simulink model "zadatak1"  (R2017b)
settings: Solver=VariableStepAuto  StartTime=0.0  StopTime=10.0  RelTol=1e-3
settings Model: Creator=HP  LastModifiedBy=HP

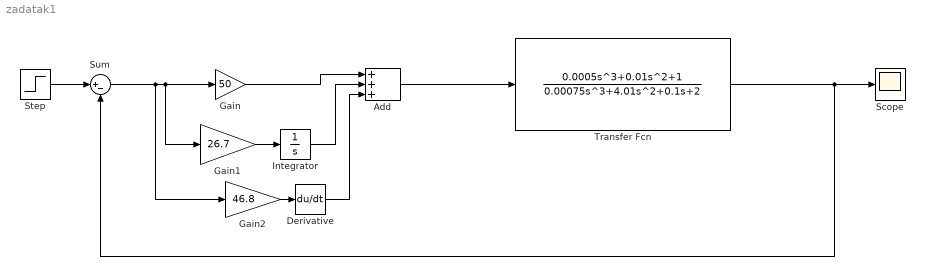
== system zadatak1 ==
  Add : Sum  Inputs=+++
  Derivative : Derivative
  Gain : Gain  Gain=50
  Gain1 : Gain  Gain=26.7
  Gain2 : Gain  Gain=46.8
  Integrator : Integrator
  Scope : Scope
  Step : Step  SampleTime=0
  Sum : Sum  Inputs=|+-
  Transfer Fcn : TransferFcn  Numerator=[0.0005 0.01 0 1]  Denominator=[0.00075 4.01 0.1 2]
  wires:
  Transfer Fcn/1 -> Sum/2, Scope/1
  Sum/1 -> Gain2/1, Gain1/1, Gain/1
  Step/1 -> Sum/1
  Gain1/1 -> Integrator/1
  Gain/1 -> Add/1
  Integrator/1 -> Add/2
  Gain2/1 -> Derivative/1
  Derivative/1 -> Add/3
  Add/1 -> Transfer Fcn/1
